simulink model "narrow_band_4fsk"  (R2022b)
settings: Solver=VariableStepAuto  StartTime=0.0  StopTime=5  RelTol=1e-3
undefined symbols (not defined in the file): DiscIntNeverNeededParam
libraries: dsparch4 x2, commsink2 x2, commfilt2 x2, dspsrcs4 x2, commchan3 x1, commrandsrc3 x1, simulink x1
settings Model: Creator=stm  LastModifiedBy=stm

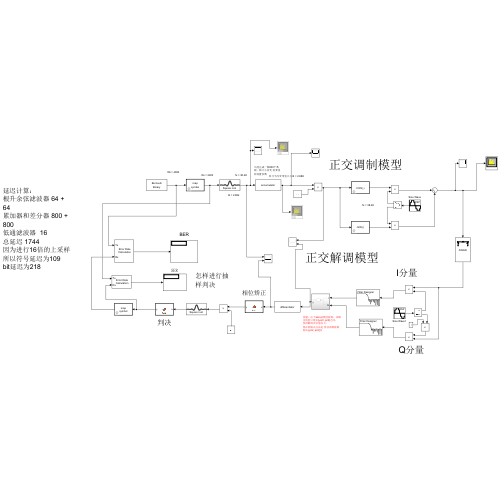
[thumbnail: Simulink's stored preview of the top-level diagram]
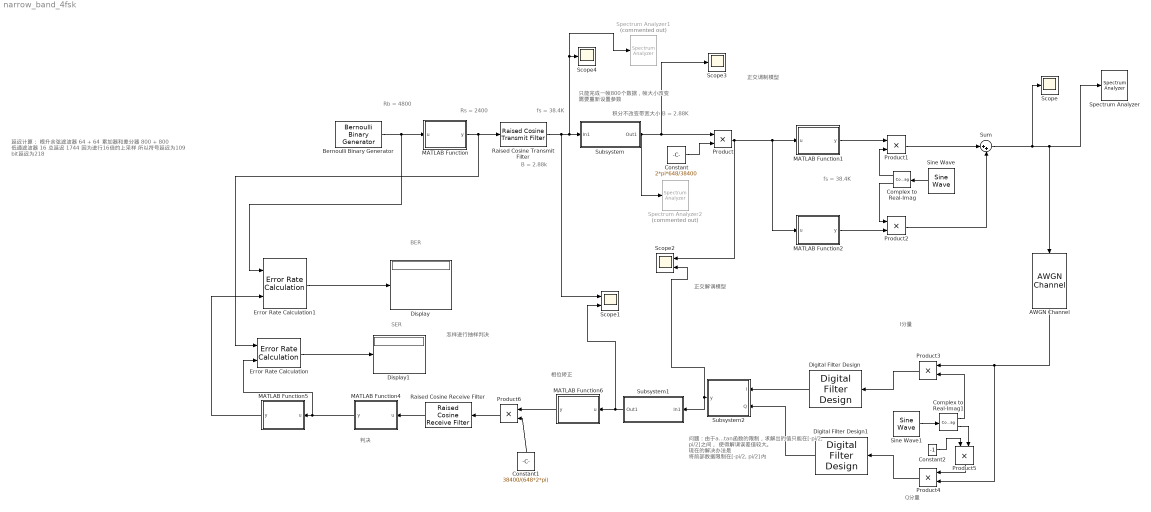
== system narrow_band_4fsk ==
  note: SER
  note: BER
  note: 积分不改变带宽大小 B = 2.88K
  note: B = 2.88k
  note: fs = 38.4K
  note: 正交调制模型
  note: 判决
  note: 问题：由于atan函数的限制，求解出的值只能在[-pi/2, pi/2]之间，
      | 使得解调误差值较大。
      | 现在的解决办法是 将前部数据限制在[-pi/2, pi/2]内
  note: I分量
  note: 相位矫正
  note: fs = 38.4K
  note: 只能完成一帧800个数据，帧大小改变 需要重新设置参数
  note: Rs = 2400
  note: 怎样进行抽样判决
  note: Rb = 4800
  note: Q分量
  note: 正交解调模型
  note: 延迟计算：
      | 根升余弦滤波器 64 + 64
      | 累加器和差分器 800 + 800
      | 低通滤波器 16
      | 总延迟 1744
      | 因为进行16倍的上采样
      | 所以符号延迟为109
      | bit延迟为218
  AWGN Channel : commchan3/AWGN Channel  InputProcessing=Columns as channels (frame based)  seed=67  noiseMode="Signal to noise ratio  (SNR)"  EbNodB=10  EsNodB=10  SNRdB=18  bitsPerSym=2  Ps=0.5  Tsym=1/2400  variance=1
  Bernoulli Binary Generator : commrandsrc3/Bernoulli Binary Generator  ProbabilityOfZero=0.5  SeedSource=Parameter  Seed=37  SampleTime=1/4800  SamplesPerFrame=100  OutputDataType=double  SimulateUsing=Interpreted execution
  Complex to Real-Imag : ComplexToRealImag
  Complex to Real-Imag1 : ComplexToRealImag
  Constant : Constant  Value=2*pi*648/38400  VectorParams1D=off
  Constant1 : Constant  Value=38400/(648*2*pi)  VectorParams1D=off
  Constant2 : Constant  Value=-1
  Digital Filter Design : dsparch4/Digital Filter Design  mwdsp_browser_bugfix_var=off
  Digital Filter Design1 : dsparch4/Digital Filter Design  mwdsp_browser_bugfix_var=off
  Display : Display
  Display1 : Display
  Error Rate Calculation : commsink2/Error Rate Calculation  N=109  st_delay=0  cp_mode=Entire frame  subframe=[]  PMode=Port  WsName=Errorsym18  RsMode2=off  stop=off  numErr=100  maxBits=1e6
  Error Rate Calculation1 : commsink2/Error Rate Calculation  N=218  st_delay=0  cp_mode=Entire frame  subframe=[]  PMode=Port  WsName=ErrorVec  RsMode2=off  stop=off  numErr=100  maxBits=1e6
  MATLAB Function : MATLAB Function  TreatAsAtomicUnit=on
  MATLAB Function1 : MATLAB Function  TreatAsAtomicUnit=on
  MATLAB Function2 : MATLAB Function  TreatAsAtomicUnit=on
  MATLAB Function4 : MATLAB Function  TreatAsAtomicUnit=on
  MATLAB Function5 : MATLAB Function  TreatAsAtomicUnit=on
  MATLAB Function6 : MATLAB Function  TreatAsAtomicUnit=on
  Product{,1..6} (7 alike) : Product
  Raised Cosine Receive Filter : commfilt2/Raised Cosine Receive Filter  filtType=Square root  R=0.2  filtSpan=8  N=16  downFactor=16  downOffset=0  filterGain=1  InputProcessing=Columns as channels (frame based)  RateOptions=Enforce single-rate processing  framing=Mute  checkCoeff=off  variableName=rcRxFilt  currentFiltSpan=10  D=5  inputOffset=0  sampMode=Mute  saveAsFlag=0  rateMode=Downsampling  checkGain=Normalized  launchFVT=on  roundingMode=Floor  overflowMode=off  coeffDataTypeStr=Inherit: Same word length as input  coeffMin=[]  coeffMax=[]  coeffLastDataTypeStr=Inherit: Same word length as input  accumDataTypeStr=Inherit: Same as product output  accumLastDataTypeStr=Inherit: Same as product output  outputDataTypeStr=Inherit: Same as accumulator  outputMin=[]  outputMax=[]  outputLastDataTypeStr=Inherit: Same as accumulator
      settings: LibrarySourceBlock=|
      | commhdlfilt/Raised Cosine
      | Receive Filter
  Raised Cosine Transmit Filter : commfilt2/Raised Cosine Transmit Filter  filtType=Square root  R=0.2  filtSpan=8  N=16  filterGain=1  InputProcessing=Columns as channels (frame based)  RateOptions=Enforce single-rate processing  framing=Mute  checkCoeff=off  variableName=rcTxFilt  checkGain=Normalized  sampMode=Mute  saveAsFlag=0  currentFiltSpan=10  D=(10)/2  launchFVT=on  roundingMode=Floor  overflowMode=off  coeffDataTypeStr=Inherit: Same word length as input  coeffMin=[]  coeffMax=[]  coeffLastDataTypeStr=Inherit: Same word length as input  outputDataTypeStr=Inherit: Same as accumulator  outputMin=[]  outputMax=[]  outputLastDataTypeStr=Inherit: Same as accumulator
  Scope : Scope
  Scope1 : Scope  NumInputPorts=2
  Scope2 : Scope  NumInputPorts=2
  Scope3 : Scope
  Scope4 : Scope
  Sine Wave : dspsrcs4/Sine Wave  Amplitude=1  Frequency=10e3  Phase=0  SampleMode=Discrete  OutComplex=Complex  CompMethod=Trigonometric fcn  TableSize=Speed  SampleTime=1/38400  SamplesPerFrame=800  ResetState=Restart at time zero  OutputFrames=off  dataType=double  wordLen=16  udDataType=sfix(16)  fracBitsMode=Best precision  numFracBits=15  OutDataTypeStr=double  LastOutDataTypeStr=double
  Sine Wave1 : dspsrcs4/Sine Wave  Amplitude=1  Frequency=10e3  Phase=0  SampleMode=Discrete  OutComplex=Complex  CompMethod=Trigonometric fcn  TableSize=Speed  SampleTime=1/38400  SamplesPerFrame=800  ResetState=Restart at time zero  OutputFrames=off  dataType=double  wordLen=16  udDataType=sfix(16)  fracBitsMode=Best precision  numFracBits=15  OutDataTypeStr=double  LastOutDataTypeStr=double
  Spectrum Analyzer : SpectrumAnalyzer
  Spectrum Analyzer1 : SpectrumAnalyzer  Commented=on
  Spectrum Analyzer2 : SpectrumAnalyzer  Commented=on
  Subsystem : Subsystem
      mask Display: disp('accumulator');
  Subsystem1 : Subsystem
      mask Display: disp('differentiator');
  Subsystem2 : Subsystem
  Sum : Sum  Inputs=|++
  wires:
  AWGN Channel/1 -> Product3/1, Product4/2
  Complex to Real-Imag1/2 -> Product5/2
  Product5/1 -> Product4/1
  MATLAB Function6/1(y) -> Product6/1
  Sum/1 -> Spectrum Analyzer/1, AWGN Channel/1, Scope/1
  Constant2/1 -> Product5/1
  Digital Filter Design/1 -> Subsystem2/1(I)
  MATLAB Function1/1(y) -> Product1/1
  Error Rate Calculation1/1 -> Display/1
  Complex to Real-Imag1/1 -> Product3/2
  Sine Wave/1 -> Complex to Real-Imag/1
  MATLAB Function5/1(y) -> Error Rate Calculation1/2
  Digital Filter Design1/1 -> Subsystem2/2(Q)
  Subsystem1/1(Out1) -> Scope1/2, MATLAB Function6/1(u)
  MATLAB Function4/1(y) -> Error Rate Calculation/2, MATLAB Function5/1(u)
  Complex to Real-Imag/2 -> Product2/1
  Subsystem2/1(y) -> Subsystem1/1(In1), Scope2/2
  Bernoulli Binary Generator/1 -> Error Rate Calculation1/1, MATLAB Function/1(u)
  Constant1/1 -> Product6/2
  Product4/1 -> Digital Filter Design1/1
  Product1/1 -> Sum/1
  Subsystem/1(Out1) -> Spectrum Analyzer2/1, Scope3/1, Product/1
  Product2/1 -> Sum/2
  Raised Cosine Receive Filter/1 -> MATLAB Function4/1(u)
  Complex to Real-Imag/1 -> Product1/2
  MATLAB Function/1(y) -> Error Rate Calculation/1, Raised Cosine Transmit Filter/1
  Raised Cosine Transmit Filter/1 -> Spectrum Analyzer1/1, Scope4/1, Subsystem/1(In1), Scope1/1
  Sine Wave1/1 -> Complex to Real-Imag1/1
  Product/1 -> Scope2/1, MATLAB Function2/1(u), MATLAB Function1/1(u)
  MATLAB Function2/1(y) -> Product2/2
  Constant/1 -> Product/2
  Product6/1 -> Raised Cosine Receive Filter/1
  Product3/1 -> Digital Filter Design/1
  Error Rate Calculation/1 -> Display1/1

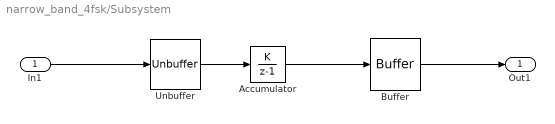
== system narrow_band_4fsk/Subsystem ==
  In1 : Inport
  Accumulator : DiscreteIntegrator  IntegratorMethod=Accumulation: Forward Euler  SampleTime=-1  ICPrevOutput=DiscIntNeverNeededParam  ICPrevScaledInput=DiscIntNeverNeededParam
  Buffer : Buffer  N=800  OutputFrames=off
  Unbuffer : Unbuffer
  Out1 : Outport
  wires:
  Accumulator/1 -> Buffer/1
  Buffer/1 -> Out1/1
  Unbuffer/1 -> Accumulator/1
  In1/1 -> Unbuffer/1

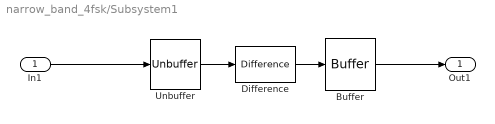
== system narrow_band_4fsk/Subsystem1 ==
  In1 : Inport
  Buffer : Buffer  N=800  OutputFrames=off
  Difference : simulink/Discrete/Difference  ICPrevInput=0.0  InputProcessing=Columns as channels (frame based)  OutMin=[]  OutMax=[]  OutDataType=fixdt(1, 16)  OutScaling=2^-10  DoSatur=off
  Unbuffer : Unbuffer
  Out1 : Outport
  wires:
  Difference/1 -> Buffer/1
  Unbuffer/1 -> Difference/1
  Buffer/1 -> Out1/1
  In1/1 -> Unbuffer/1

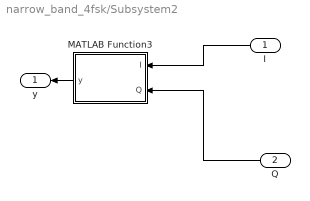
== system narrow_band_4fsk/Subsystem2 ==
  I : Inport
  Q : Inport  Port=2
  MATLAB Function3 : MATLAB Function  TreatAsAtomicUnit=on
  y : Outport
  wires:
  I/1 -> MATLAB Function3/1(I)
  Q/1 -> MATLAB Function3/2(Q)
  MATLAB Function3/1(y) -> y/1

== matlab function narrow_band_4fsk/MATLAB Function ==
  data: u input; y output
function y = fcn(u)

len = length(u);
y = zeros(len/2, 1);
for i = 1:2:len-1
    id = (i-1)/2 + 1;
    switch(u(i))

        case 1
            if(u(i+1) == 1) 
                y(id) = 3;
            else 
                y(id) = 1;
            end

        case 0
            if(u(i+1) == 1) 
                y(id) = -1;
            else 
                y(id) = -3;
            end

    end


end

== matlab function narrow_band_4fsk/MATLAB Function2 ==
  data: u input; y output
function y = fcn(u)

y = -sin(u);

== matlab function narrow_band_4fsk/Subsystem2/MATLAB Function3 ==
  data: I input; Q input; y output
function y = fcn(I,Q)

y = atan(Q./I);

== matlab function narrow_band_4fsk/MATLAB Function4 ==
  data: u input; y output
function y = fcn(u)

u(u >= 2) = 3;
u(u < -2) = -3;
u(u >= 0 & u < 2) = 1;
u(u < 0 & u >=-2) = -1;

y = u;

== matlab function narrow_band_4fsk/MATLAB Function5 ==
  data: u input; y output
function y = fcn(u)

len = length(u);
y = zeros(len*2, 1);
for i = 1:len
    id = 2*i;
    switch(u(i))

        case -3
         y(id-1) = 0;
         y(id) = 0;

        case -1
         y(id-1) = 0;
         y(id) = 1;
        case 1
         y(id-1) = 1;
         y(id) = 0;
        case 3
         y(id-1) = 1;
         y(id) = 1;
    end


end

== matlab function narrow_band_4fsk/MATLAB Function6 ==
  data: u input; y output
function y = fcn(u)

id1 = u > pi/2;

id2 = u < -pi/2;

u(id1) = u(id1) - pi;
u(id2) = u(id2) + pi;

y = u;

== matlab function narrow_band_4fsk/MATLAB Function1 ==
  data: u input; y output
function y = fcn(u)

y = cos(u);
